simulink model "SystemsmModelling_ModifyAirCon"  (R2020a)
settings: Solver=ode23t  StartTime=0.0  StopTime=20000  MaxStep=2000.0  RelTol=1e-3
values from neighbouring files (symbols this model uses):
  InitialTemp = 300    [Setup.m]
undefined symbols (not defined in the file or in its folder): building_height, building_length, building_width, duct_area, environment_temperature, fan_flow_rate_table, fan_setting_table, floor_conductivity, floor_heat_transfer_coeff_internal, floor_thickness, ground_temperature, initial_temperature, roof_conductivity, roof_density, roof_heat_transfer_coeff_external, roof_heat_transfer_coeff_internal, roof_specific_heat, roof_thickness, sigbuilder_block, wall_conductivity, wall_density, wall_heat_transfer_coeff_external, wall_heat_transfer_coeff_internal, wall_specific_heat, wall_thickness
libraries: fl_lib x78, nesl_utility x16
(part 1 of 3)
settings Model: Creator=denni  LastModifiedBy=denni

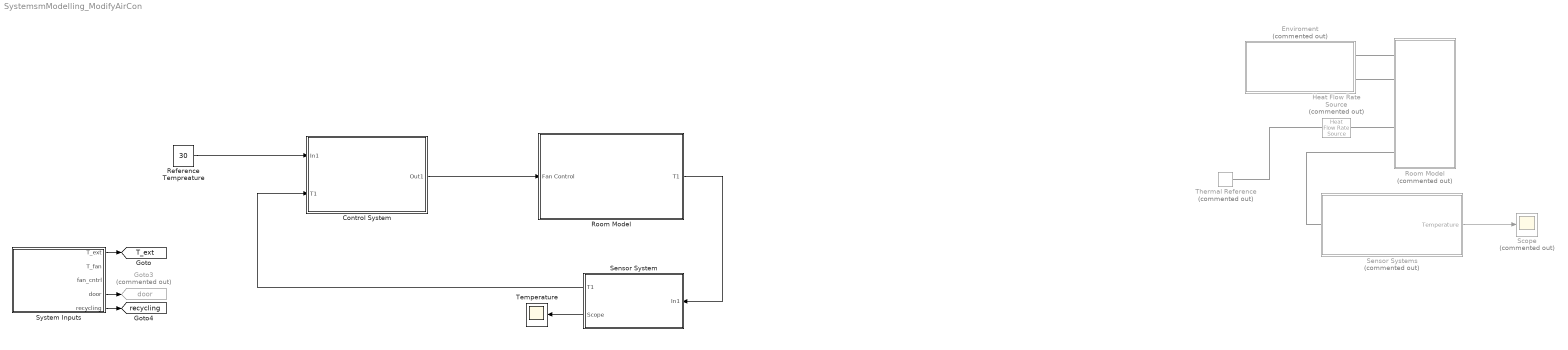
== system SystemsmModelling_ModifyAirCon ==
  Control System : Subsystem
  Enviroment : Subsystem  Commented=on
  Goto3 : Goto  Commented=on  GotoTag=door  TagVisibility=global
  Heat Flow Rate Source : fl_lib/Thermal/Thermal Sources/Heat Flow Rate Source  Commented=on  heat_flow=10 W
      settings: SourceProductBaseCode=SS  InternalSimscapePortConfiguration="{\"Bottom\":[],\"Left\":[{\"id\":\"B\",\"label\":\"B\",\"type\":\"foundation.thermal.thermal\"}],\"Right\":[{\"id\":\"A\",\"label\":\"A\",\"type\":\"foundation.thermal.thermal\"}],\"Top\":[]}"
  "Reference Tempreature " : Constant  Value=30
  Room Model : Subsystem  Commented=on
  "Room Model " : Subsystem
  Scope : Scope  Commented=on
  Sensor System : Subsystem
  Sensor Systems : Subsystem  Commented=on
  System Inputs : Subsystem  Tag=STV Subsys  LoadFcn=sigbuilder_block('load');  StartFcn=sigbuilder_block('start');  StopFcn=sigbuilder_block('stop');  ClipboardFcn=sigbuilder_block('clipboard');  mask(Sigbuilder block){tuvar=[0:10]}
      mask help: Simulink:masks:SigbuilderBlock_MD
      mask init:
      | if ~strcmp(get_param(bdroot(gcbh),'SimulationStatus'),'stopped') tuvar = sigbuilder_block('maskInit'); end
      settings: CopyFcn=sigbuilder_block('copy');  DeleteFcn=sigbuilder_block('delete');  ModelCloseFcn=sigbuilder_block('modelClose');  PreSaveFcn=sigbuilder_block('preSave');  PauseFcn=sigbuilder_block('pause');  ContinueFcn=sigbuilder_block('continue');  NameChangeFcn=sigbuilder_block('namechange');  OpenFcn=sigbuilder_block('open',[334.8 172.8 550.8 361.2 ]);  CloseFcn=sigbuilder_block('close');
      mask Display: plot(0, 0, 100, 100,[2, 2, 32, 32, 2], [68, 8, 8, 68, 68],[32, 2], [38, 38], [32, 19, 2],[53, 60, 44], [32, 17, 17, 2],[16, 16, 31, 31]);txt = getActiveGroup(gcbh);text(2, 100, txt,'verticalAlignment', 'top');
  Temperature : Scope
  Thermal Reference : fl_lib/Thermal/Thermal Elements/Thermal Reference  Commented=on
  tag scope: T_ext=global, recycling=global
  wires:
  Sensor Systems/1("Temperature ") -> Scope/1
  System Inputs/5(recycling) -> [recycling]
  System Inputs/4(door) -> Goto3/1
  System Inputs/1(T_ext) -> [T_ext]
  "Reference Tempreature "/1 -> Control System/1(In1)
  Sensor System/1(T1) -> Control System/2(T1)
  Sensor System/2(Scope) -> Temperature/1
  Control System/1(Out1) -> "Room Model "/1(Fan Control)
  "Room Model "/1(T1) -> Sensor System/1(In1)
  connections:
  Room Model/LConn1 -- Enviroment/LConn1
  Enviroment/LConn2 -- Room Model/LConn2
  Sensor Systems/LConn1 -- Room Model/LConn5
  Heat Flow Rate Source/LConn1 -- Room Model/LConn4
  Heat Flow Rate Source/RConn1 -- Thermal Reference/LConn1

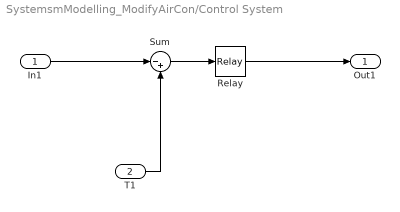
== system SystemsmModelling_ModifyAirCon/Control System ==
  In1 : Inport
  T1 : Inport  Port=2
  Relay : Relay  OnSwitchValue=2  OffSwitchValue=-2
  Sum : Sum  Inputs=|-+
  Out1 : Outport
  wires:
  Sum/1 -> Relay/1
  Relay/1 -> Out1/1
  T1/1 -> Sum/2
  In1/1 -> Sum/1

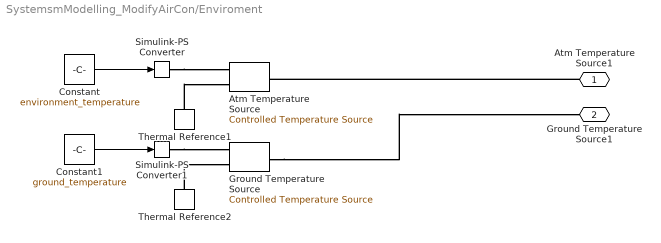
== system SystemsmModelling_ModifyAirCon/Enviroment ==
  Atm Temperature Source : fl_lib/Thermal/Thermal Sources/Controlled Temperature Source
  Constant : Constant  Value=environment_temperature
  Constant1 : Constant  Value=ground_temperature
  Ground Temperature Source : fl_lib/Thermal/Thermal Sources/Controlled Temperature Source
  Simulink-PS Converter : nesl_utility/Simulink-PS Converter  PhysicalDomain=network_engine_domain  SubClassName=ps_input  LeftPortType=input  RightPortType=output  PseudoPeriodic=off  Frequencies=[]  NoiseDistribution=none  NoiseParameters=[]  Unit=1  AffineConversion=off  FilteringAndDerivatives=provide  SimscapeFilterOrder=1  InputFilterTimeConstant=0.001  UdotUserProvided=0
  Simulink-PS Converter1 : nesl_utility/Simulink-PS Converter  PhysicalDomain=network_engine_domain  SubClassName=ps_input  LeftPortType=input  RightPortType=output  PseudoPeriodic=off  Frequencies=[]  NoiseDistribution=none  NoiseParameters=[]  Unit=1  AffineConversion=off  FilteringAndDerivatives=provide  SimscapeFilterOrder=1  InputFilterTimeConstant=0.001  UdotUserProvided=0
  Thermal Reference1 : fl_lib/Thermal/Thermal Elements/Thermal Reference
  Thermal Reference2 : fl_lib/Thermal/Thermal Elements/Thermal Reference
  Atm Temperature Source1 : PMIOPort  Side=Left
  Ground Temperature Source1 : PMIOPort  Port=2  Side=Left
  wires:
  Constant/1 -> Simulink-PS Converter/1
  Constant1/1 -> Simulink-PS Converter1/1
  connections:
  Thermal Reference2/LConn1 -- Ground Temperature Source/RConn2
  Thermal Reference1/LConn1 -- Atm Temperature Source/RConn2
  Simulink-PS Converter1/RConn1 -- Ground Temperature Source/RConn1
  Ground Temperature Source/LConn1 -- Ground Temperature Source1/RConn1
  Atm Temperature Source1/RConn1 -- Atm Temperature Source/LConn1
  Simulink-PS Converter/RConn1 -- Atm Temperature Source/RConn1

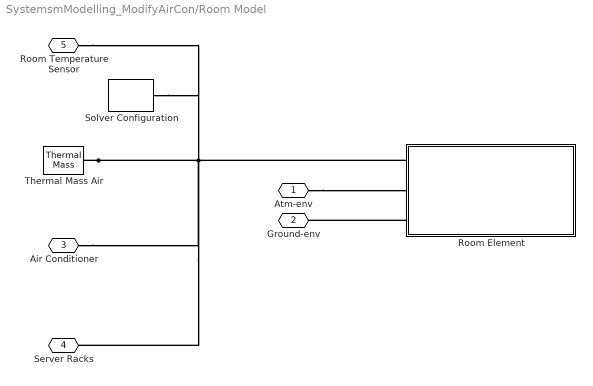
== system SystemsmModelling_ModifyAirCon/Room Model ==
  "Room Element " : Subsystem
  Solver Configuration : nesl_utility/Solver Configuration  PhysicalDomain=network_engine_domain  SubClassName=solver  LeftPortType=input  RightPortType=generic  Tones=[]  Harmonics=[]  SimulateNoise=off  Profile=off  UseLocalSampling=off  EnableSwitchedLinearOptims=on  FrequencyDomain=off  UseCCode=off  RelTol=0.001  AbsTol=1e-06  MinStep=1e-09  ToWorkspace=off  RevertToSquareIcSolve=off  NumHomotopyIterations=100  PhasorMode=off  PhasorModeNumHarmonics=1  DoDC=off  ResidualTolerance=1e-09  UseLocalSolver=off  LocalSolverChoice=NE_BACKWARD_EULER_ADVANCER  LocalSolverSampleTime=0.001  DoFixedCost=off  MaxNonlinIter=3  MaxModeIter=2  LinearAlgebra=auto  EquationFormulation=NE_TIME_EF  DelaysMemoryBudget=1024  AutomaticFiltering=on  FilteringTimeConstant=0.001  PartitionStorageMethod=AS_NEEDED  PartitionMemoryBudget=1024  PartitionMethod=ROBUST
  Thermal Mass Air : fl_lib/Thermal/Thermal Elements/Thermal Mass  mass=1 kg  sp_heat=1012 J/kg/K  T_specify=off  T_priority=High  T=300 K  T_nominal_specify=off  T_nominal_unit=K  T_nominal_value=1  Q_specify=off  Q_priority=None  Q=0 W  Q_nominal_specify=off  Q_nominal_unit=W  Q_nominal_value=1
  Atm-env : PMIOPort  Side=Left
  Ground-env : PMIOPort  Port=2  Side=Left
  Air Conditioner : PMIOPort  Port=3  Side=Left
  Server Racks : PMIOPort  Port=4  Side=Left
  "Room Temperature Sensor " : PMIOPort  Port=5  Side=Left
  connections:
  Thermal Mass Air/LConn1 -- Server Racks/RConn1 -- Air Conditioner/RConn1 -- "Room Temperature Sensor "/RConn1 -- Solver Configuration/RConn1 -- "Room Element "/LConn1
  Atm-env/RConn1 -- "Room Element "/LConn2
  "Room Element "/LConn3 -- Ground-env/RConn1

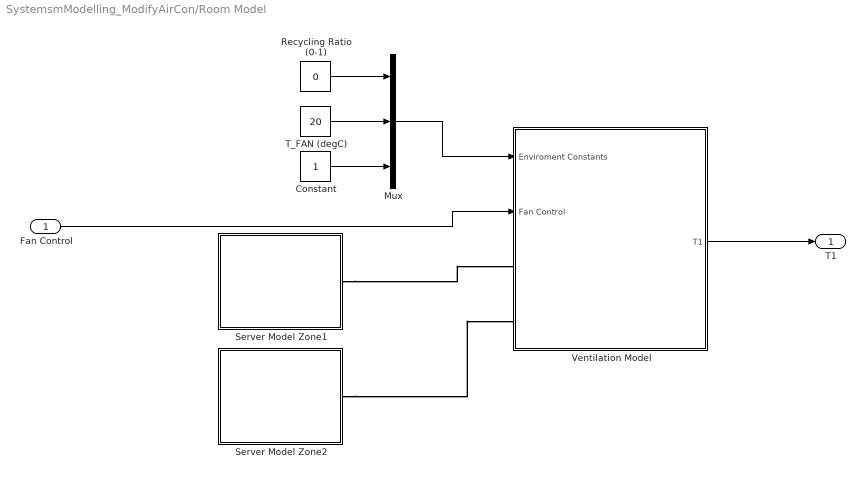
== system SystemsmModelling_ModifyAirCon/Room Model  ==
  Fan Control : Inport
  Constant : Constant
  Mux : Mux  Inputs=3
  Recycling Ratio (0-1) : Constant  Value=0
  Server Model Zone1 : Subsystem
  Server Model Zone2 : Subsystem
  T_FAN (degC) : Constant  Value=20
  Ventilation Model : Subsystem
  T1 : Outport
  wires:
  Constant/1 -> Mux/3
  Recycling Ratio (0-1)/1 -> Mux/1
  T_FAN (degC)/1 -> Mux/2
  Mux/1 -> Ventilation Model/1(Enviroment Constants)
  Fan Control/1 -> Ventilation Model/2(Fan Control)
  Ventilation Model/1(T1) -> T1/1
  connections:
  Server Model Zone1/LConn1 -- Ventilation Model/LConn1
  Server Model Zone2/LConn1 -- Ventilation Model/LConn2

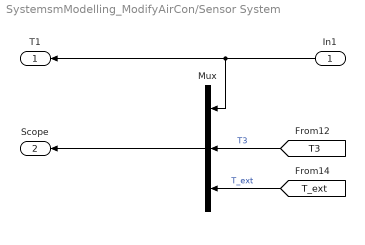
== system SystemsmModelling_ModifyAirCon/Sensor System ==
  In1 : Inport
  Mux : Mux  Inputs=3
  T1 : Outport
  Scope : Outport  Port=2
  wires:
  [T3] -> Mux/2  "T3"
  Mux/1 -> Scope/1
  [T_ext] -> Mux/3  "T_ext"
  In1/1 -> Mux/1, T1/1

== system SystemsmModelling_ModifyAirCon/Sensor Systems ==
  PS-Simulink Converter : nesl_utility/PS-Simulink Converter  PhysicalDomain=network_engine_domain  SubClassName=ps_output  LeftPortType=input  RightPortType=output  PseudoPeriodic=off  Frequencies=[]  Unit=inherit  AffineConversion=off
  Room Temperature Sensor : fl_lib/Thermal/Thermal Sensors/Temperature Sensor
  Thermal Reference : fl_lib/Thermal/Thermal Elements/Thermal Reference
  Room Temperature Sensor1 : PMIOPort  Side=Left
  "Temperature " : Outport
  wires:
  PS-Simulink Converter/1 -> "Temperature "/1
  connections:
  PS-Simulink Converter/LConn1 -- Room Temperature Sensor/RConn2
  Thermal Reference/LConn1 -- Room Temperature Sensor/RConn1
  Room Temperature Sensor/LConn1 -- Room Temperature Sensor1/RConn1

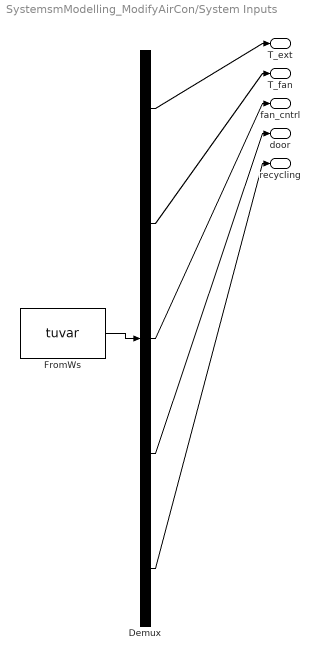
== system SystemsmModelling_ModifyAirCon/System Inputs ==
  Demux : Demux  Tag=STV Demux  Outputs=5
      settings: DisplayOption=none
  FromWs : FromWorkspace  Tag=STV FromWs  VariableName=tuvar
      SigBuilderData=|
      | common.afterFinalStr = 'Extrapolate'
      | common.sampleTime = 0
      | dataSet(1).timeRange = [0 100000]
      | dataSet(1).name = 'Fan Control'
      | dataSet(2).timeRange = [0 100000]
      | dataSet(2).name = 'Fan Temperature'
      | dataSet(3).timeRange = [0 100000]
      | dataSet(3).name = 'Disturbances'
      | sbobj.Groups(1).Name = 'Fan Control'
      | sbobj.Groups(1).Signals(1).Name = 'T_ext'
      | sbobj.Groups(1).Signals(1).XData = [0 100000]
      | sbobj.Groups(1).Signals(1).YData = [35 35]
      | sbobj.Groups(1).Signals(2).Name = 'T_fan'
      | sbobj.Groups(1).Signals(2).XData = [0 100000]
      | sbobj.Groups(1).Signals(2).YData = [20.05 20.05]
      | sbobj.Groups(1).Signals(3).Name = 'fan_cntrl'
      | sbobj.Groups(1).Signals(3).XData = [0 20000 20000 40000 60000 80000 100000]
      | sbobj.Groups(1).Signals(3).YData = [1.1 1.1 1.04 1.04 1.04 1.04 1.04]
      | sbobj.Groups(1).Signals(4).Name = 'door'
      | sbobj.Groups(1).Signals(4).XData = [0 100000]
      | sbobj.Groups(1).Signals(4).YData = [0 0]
      | sbobj.Groups(1).Signals(5).Name = 'recycling'
      | sbobj.Groups(1).Signals(5).XData = [0 100000]
      | sbobj.Groups(1).Signals(5).YData = [0 0]
      | sbobj.Groups(1).TimeRange = [0 100000]
      | sbobj.Groups(2).Name = 'Fan Temperature'
      | sbobj.Groups(2).Signals(1).Name = 'T_ext'
      | sbobj.Groups(2).Signals(1).XData = [0 100000]
      | sbobj.Groups(2).Signals(1).YData = [35 35]
      | sbobj.Groups(2).Signals(2).Name = 'T_fan'
      | sbobj.Groups(2).Signals(2).XData = [0 20000 20000 40000 40000 60000 60000 80000 80000 100000]
      | sbobj.Groups(2).Signals(2).YData = [20 20 15 15 20 20 35 35 20 20]
      | sbobj.Groups(2).Signals(3).Name = 'fan_cntrl'
      | sbobj.Groups(2).Signals(3).XData = [0 100000]
      | sbobj.Groups(2).Signals(3).YData = [1 1]
      | sbobj.Groups(2).Signals(4).Name = 'door'
      | sbobj.Groups(2).Signals(4).XData = [0 100000]
      | sbobj.Groups(2).Signals(4).YData = [0 0]
      | sbobj.Groups(2).Signals(5).Name = 'recycling'
      | sbobj.Groups(2).Signals(5).XData = [0 100000]
      | sbobj.Groups(2).Signals(5).YData = [0 0]
      | sbobj.Groups(2).TimeRange = [0 100000]
      | sbobj.Groups(3).Name = 'Disturbances'
      | sbobj.Groups(3).Signals(1).Name = 'T_ext'
      | sbobj.Groups(3).Signals(1).XData = [0 100000]
      | sbobj.Groups(3).Signals(1).YData = [35 35]
      | sbobj.Groups(3).Signals(2).Name = 'T_fan'
      | sbobj.Groups(3).Signals(2).XData = [0 100000]
      | sbobj.Groups(3).Signals(2).YData = [20 20]
      | sbobj.Groups(3).Signals(3).Name = 'fan_cntrl'
      | sbobj.Groups(3).Signals(3).XData = [0 100000]
      | sbobj.Groups(3).Signals(3).YData = [1 1]
      | sbobj.Groups(3).Signals(4).Name = 'door'
      | sbobj.Groups(3).Signals(4).XData = [0 20000 30000 40000 100000]
      | sbobj.Groups(3).Signals(4).YData = [0 0 1 0 0]
      | sbobj.Groups(3).Signals(5).Name = 'recycling'
      | sbobj.Groups(3).Signals(5).XData = [0 60000 60000 80000 80000 100000]
      | sbobj.Groups(3).Signals(5).YData = [0 0 0.5 0.5 0 0]
      | sbobj.Groups(3).TimeRange = [0 100000]
  T_ext : Outport  Tag=STV Outport  VectorParamsAs1DForOutWhenUnconnected=off
  T_fan : Outport  Tag=STV Outport  Port=2  VectorParamsAs1DForOutWhenUnconnected=off
  fan_cntrl : Outport  Tag=STV Outport  Port=3  VectorParamsAs1DForOutWhenUnconnected=off
  door : Outport  Tag=STV Outport  Port=4  VectorParamsAs1DForOutWhenUnconnected=off
  recycling : Outport  Tag=STV Outport  Port=5  VectorParamsAs1DForOutWhenUnconnected=off
  wires:
  FromWs/1 -> Demux/1
  Demux/1 -> T_ext/1
  Demux/2 -> T_fan/1
  Demux/3 -> fan_cntrl/1
  Demux/4 -> door/1
  Demux/5 -> recycling/1

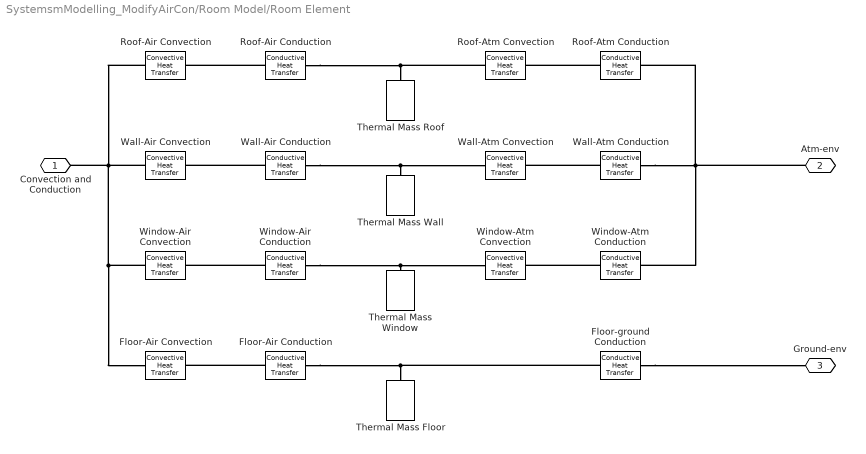
== system SystemsmModelling_ModifyAirCon/Room Model/Room Element  ==
  " Wall-Air Conduction" : fl_lib/Thermal/Thermal Elements/Conductive Heat Transfer  area=375 m^2  thickness=0.2 m  th_cond=0.15 W/(m*K)  T_specify=off  T_priority=None  T=0 K  T_nominal_specify=off  T_nominal_unit=K  T_nominal_value=1  Q_specify=off  Q_priority=None  Q=0 W  Q_nominal_specify=off  Q_nominal_unit=W  Q_nominal_value=1
  " Wall-Atm Conduction" : fl_lib/Thermal/Thermal Elements/Conductive Heat Transfer  area=375 m^2  thickness=0.2 m  th_cond=0.15 W/(m*K)  T_specify=off  T_priority=None  T=0 K  T_nominal_specify=off  T_nominal_unit=K  T_nominal_value=1  Q_specify=off  Q_priority=None  Q=0 W  Q_nominal_specify=off  Q_nominal_unit=W  Q_nominal_value=1
  " Window-Air Conduction" : fl_lib/Thermal/Thermal Elements/Conductive Heat Transfer  area=25 m^2  thickness=0.2 m  th_cond=0.96 W/(m*K)  T_specify=off  T_priority=None  T=0 K  T_nominal_specify=off  T_nominal_unit=K  T_nominal_value=1  Q_specify=off  Q_priority=None  Q=0 W  Q_nominal_specify=off  Q_nominal_unit=W  Q_nominal_value=1
  " Window-Atm Conduction" : fl_lib/Thermal/Thermal Elements/Conductive Heat Transfer  area=25 m^2  thickness=0.2 m  th_cond=0.96 W/(m*K)  T_specify=off  T_priority=None  T=0 K  T_nominal_specify=off  T_nominal_unit=K  T_nominal_value=1  Q_specify=off  Q_priority=None  Q=0 W  Q_nominal_specify=off  Q_nominal_unit=W  Q_nominal_value=1
  Floor-Air Conduction : fl_lib/Thermal/Thermal Elements/Conductive Heat Transfer  area=25 m^2  thickness=0.2 m  th_cond=0.96 W/(m*K)  T_specify=off  T_priority=None  T=0 K  T_nominal_specify=off  T_nominal_unit=K  T_nominal_value=1  Q_specify=off  Q_priority=None  Q=0 W  Q_nominal_specify=off  Q_nominal_unit=W  Q_nominal_value=1
  Floor-Air Convection : fl_lib/Thermal/Thermal Elements/Convective Heat Transfer  area=20 m^2  heat_tr_coeff=3.3 W/(m^2 * K)  T_specify=off  T_priority=None  T=0 K  T_nominal_specify=off  T_nominal_unit=K  T_nominal_value=1  Q_specify=off  Q_priority=None  Q=0 W  Q_nominal_specify=off  Q_nominal_unit=W  Q_nominal_value=1
  Floor-ground Conduction : fl_lib/Thermal/Thermal Elements/Conductive Heat Transfer  area=25 m^2  thickness=0.2 m  th_cond=0.96 W/(m*K)  T_specify=off  T_priority=None  T=0 K  T_nominal_specify=off  T_nominal_unit=K  T_nominal_value=1  Q_specify=off  Q_priority=None  Q=0 W  Q_nominal_specify=off  Q_nominal_unit=W  Q_nominal_value=1
  Roof-Air Conduction : fl_lib/Thermal/Thermal Elements/Conductive Heat Transfer  area=100 m^2  thickness=0.2 m  th_cond=0.12 W/(m*K)  T_specify=off  T_priority=None  T=0 K  T_nominal_specify=off  T_nominal_unit=K  T_nominal_value=1  Q_specify=off  Q_priority=None  Q=0 W  Q_nominal_specify=off  Q_nominal_unit=W  Q_nominal_value=1
  Roof-Air Convection : fl_lib/Thermal/Thermal Elements/Convective Heat Transfer  area=100 m^2  heat_tr_coeff=20 W/(m^2 * K)  T_specify=off  T_priority=None  T=0 K  T_nominal_specify=off  T_nominal_unit=K  T_nominal_value=1  Q_specify=off  Q_priority=None  Q=0 W  Q_nominal_specify=off  Q_nominal_unit=W  Q_nominal_value=1
  Roof-Atm Conduction : fl_lib/Thermal/Thermal Elements/Conductive Heat Transfer  area=100 m^2  thickness=0.2 m  th_cond=0.12 W/(m*K)  T_specify=off  T_priority=None  T=0 K  T_nominal_specify=off  T_nominal_unit=K  T_nominal_value=1  Q_specify=off  Q_priority=None  Q=0 W  Q_nominal_specify=off  Q_nominal_unit=W  Q_nominal_value=1
  Roof-Atm Convection : fl_lib/Thermal/Thermal Elements/Convective Heat Transfer  area=100 m^2  heat_tr_coeff=20 W/(m^2 * K)  T_specify=off  T_priority=None  T=0 K  T_nominal_specify=off  T_nominal_unit=K  T_nominal_value=1  Q_specify=off  Q_priority=None  Q=0 W  Q_nominal_specify=off  Q_nominal_unit=W  Q_nominal_value=1
  Thermal Mass Floor : fl_lib/Thermal/Thermal Elements/Thermal Mass  mass=48 kg  sp_heat=840.7 J/kg/K  T_specify=on  T_priority=High  T=InitialTemp K  T_nominal_specify=off  T_nominal_unit=K  T_nominal_value=1  Q_specify=off  Q_priority=None  Q=0 W  Q_nominal_specify=off  Q_nominal_unit=W  Q_nominal_value=1
  Thermal Mass Roof : fl_lib/Thermal/Thermal Elements/Thermal Mass  mass=48 kg  sp_heat=853.7 J/kg/K  T_specify=on  T_priority=High  T=InitialTemp K  T_nominal_specify=off  T_nominal_unit=K  T_nominal_value=1  Q_specify=off  Q_priority=None  Q=0 W  Q_nominal_specify=off  Q_nominal_unit=W  Q_nominal_value=1
  Thermal Mass Wall : fl_lib/Thermal/Thermal Elements/Thermal Mass  mass=180 kg  sp_heat=868.2 J/kg/K  T_specify=on  T_priority=High  T=InitialTemp K  T_nominal_specify=off  T_nominal_unit=K  T_nominal_value=1  Q_specify=off  Q_priority=None  Q=0 W  Q_nominal_specify=off  Q_nominal_unit=W  Q_nominal_value=1
  Thermal Mass Window : fl_lib/Thermal/Thermal Elements/Thermal Mass  mass=11 kg  sp_heat=840 J/kg/K  T_specify=on  T_priority=High  T=InitialTemp K  T_nominal_specify=off  T_nominal_unit=K  T_nominal_value=1  Q_specify=off  Q_priority=None  Q=0 W  Q_nominal_specify=off  Q_nominal_unit=W  Q_nominal_value=1
  Wall-Air Convection : fl_lib/Thermal/Thermal Elements/Convective Heat Transfer  area=375 m^2  heat_tr_coeff=20 W/(m^2 * K)  T_specify=off  T_priority=None  T=0 K  T_nominal_specify=off  T_nominal_unit=K  T_nominal_value=1  Q_specify=off  Q_priority=None  Q=0 W  Q_nominal_specify=off  Q_nominal_unit=W  Q_nominal_value=1
  Wall-Atm Convection : fl_lib/Thermal/Thermal Elements/Convective Heat Transfer  area=375 m^2  heat_tr_coeff=20 W/(m^2 * K)  T_specify=off  T_priority=None  T=0 K  T_nominal_specify=off  T_nominal_unit=K  T_nominal_value=1  Q_specify=off  Q_priority=None  Q=0 W  Q_nominal_specify=off  Q_nominal_unit=W  Q_nominal_value=1
  Window-Air Convection : fl_lib/Thermal/Thermal Elements/Convective Heat Transfer  area=25 m^2  heat_tr_coeff=3.3 W/(m^2 * K)  T_specify=off  T_priority=None  T=0 K  T_nominal_specify=off  T_nominal_unit=K  T_nominal_value=1  Q_specify=off  Q_priority=None  Q=0 W  Q_nominal_specify=off  Q_nominal_unit=W  Q_nominal_value=1
  Window-Atm Convection : fl_lib/Thermal/Thermal Elements/Convective Heat Transfer  area=25 m^2  heat_tr_coeff=3.3 W/(m^2 * K)  T_specify=off  T_priority=None  T=0 K  T_nominal_specify=off  T_nominal_unit=K  T_nominal_value=1  Q_specify=off  Q_priority=None  Q=0 W  Q_nominal_specify=off  Q_nominal_unit=W  Q_nominal_value=1
  Convection and Conduction : PMIOPort  Side=Left
  Atm-env : PMIOPort  Port=2  Side=Left
  Ground-env : PMIOPort  Port=3  Side=Left
  connections:
  " Window-Atm Conduction"/RConn1 -- Window-Atm Convection/LConn1
  Floor-ground Conduction/LConn1 -- Ground-env/RConn1
  Roof-Air Conduction/RConn1 -- Roof-Air Convection/LConn1
  Floor-Air Conduction/LConn1 -- Floor-ground Conduction/RConn1 -- Thermal Mass Floor/LConn1
  " Wall-Atm Conduction"/LConn1 -- Atm-env/RConn1 -- Roof-Atm Conduction/LConn1 -- " Window-Atm Conduction"/LConn1
  Roof-Air Convection/RConn1 -- Convection and Conduction/RConn1 -- Window-Air Convection/RConn1 -- Floor-Air Convection/RConn1 -- Wall-Air Convection/RConn1
  Roof-Atm Convection/RConn1 -- Roof-Air Conduction/LConn1 -- Thermal Mass Roof/LConn1
  Roof-Atm Conduction/RConn1 -- Roof-Atm Convection/LConn1
  " Wall-Air Conduction"/LConn1 -- Wall-Atm Convection/RConn1 -- Thermal Mass Wall/LConn1
  " Window-Air Conduction"/LConn1 -- Window-Atm Convection/RConn1 -- Thermal Mass Window/LConn1
  " Wall-Atm Conduction"/RConn1 -- Wall-Atm Convection/LConn1
  " Wall-Air Conduction"/RConn1 -- Wall-Air Convection/LConn1
  " Window-Air Conduction"/RConn1 -- Window-Air Convection/LConn1
  Floor-Air Conduction/RConn1 -- Floor-Air Convection/LConn1

== system SystemsmModelling_ModifyAirCon/Room Model /Server Model Zone1 ==
  Heat Flow Rate Source1 : fl_lib/Thermal/Thermal Sources/Heat Flow Rate Source  heat_flow=500 W
      settings: SourceProductBaseCode=SS  InternalSimscapePortConfiguration="{\"Bottom\":[],\"Left\":[{\"id\":\"B\",\"label\":\"B\",\"type\":\"foundation.thermal.thermal\"}],\"Right\":[{\"id\":\"A\",\"label\":\"A\",\"type\":\"foundation.thermal.thermal\"}],\"Top\":[]}"
  Thermal Reference1 : fl_lib/Thermal/Thermal Elements/Thermal Reference
  Heat Flow Rate Source2 : PMIOPort  Side=Left
  connections:
  Heat Flow Rate Source1/RConn1 -- Thermal Reference1/LConn1
  Heat Flow Rate Source1/LConn1 -- Heat Flow Rate Source2/RConn1

== system SystemsmModelling_ModifyAirCon/Room Model /Server Model Zone2 ==
  Heat Flow Rate Source1 : fl_lib/Thermal/Thermal Sources/Heat Flow Rate Source  heat_flow=500 W
      settings: SourceProductBaseCode=SS  InternalSimscapePortConfiguration="{\"Bottom\":[],\"Left\":[{\"id\":\"B\",\"label\":\"B\",\"type\":\"foundation.thermal.thermal\"}],\"Right\":[{\"id\":\"A\",\"label\":\"A\",\"type\":\"foundation.thermal.thermal\"}],\"Top\":[]}"
  Thermal Reference1 : fl_lib/Thermal/Thermal Elements/Thermal Reference
  Heat Flow Rate Source2 : PMIOPort  Side=Left
  connections:
  Heat Flow Rate Source1/RConn1 -- Thermal Reference1/LConn1
  Heat Flow Rate Source1/LConn1 -- Heat Flow Rate Source2/RConn1
